simulink model "BiCopter_Height"  (R2016a)
settings: Solver=VariableStepAuto  StartTime=0.0  StopTime=10.0  RelTol=1e-3
values from neighbouring files (symbols this model uses):
  A = [0 1 ... (first row only)    [BiCopter_HeightOnly.m]    (also in BiCopter_script.m = [0 0 0 1 0 0)
  B = [0; 2/m]    [BiCopter_HeightOnly.m]    (also in BiCopter_script.m = [0 0)
  C = eye(2)    [BiCopter_HeightOnly.m]    (also in BiCopter_script.m = zeros(6,6))
  D = [0; 0]    [BiCopter_HeightOnly.m]    (also in BiCopter_script.m = zeros(6,2))
  K = place(A,B,p)    [BiCopter_HeightOnly.m]    (also in BiCopter_script.m)
  Kr = -inv( (C-D*K)*inv(A-B*K)*B - D)    [BiCopter_HeightOnly.m]    (also in BiCopter_script.m = -inv( (C)*inv(A-B*K)*B))
  r = 2    [BiCopter_HeightOnly.m]    (also in BiCopter_script.m = [0; 10])
settings Model: Creator=Austin  LastModifiedBy=Austin

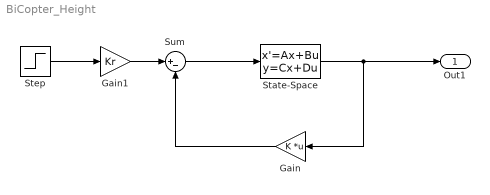
== system BiCopter_Height ==
  Gain : Gain  Gain=K  Multiplication=Matrix(K*u)
  Gain1 : Gain  Gain=Kr
  State-Space : StateSpace  A=A  B=B  C=C  D=D  X0=0
  Step : Step  After=r  SampleTime=0
  Sum : Sum  Inputs=|+-
  Out1 : Outport
  wires:
  Gain/1 -> Sum/2
  State-Space/1 -> Gain/1, Out1/1
  Sum/1 -> State-Space/1
  Gain1/1 -> Sum/1
  Step/1 -> Gain1/1
